simulink model "fromWorkSpace_TestGen6"  (R2017b)
settings: Solver=FixedStepDiscrete  StartTime=0.0  StopTime=10.0  RelTol=1e-3
model workspace (MAT data in the model file):
  X_matrix = [0 0.2 0.4 0.6 0.8 1 1.2 1.4 1.6 1.8 2 2.2 ... (200 elements, 50x4)]
undefined symbols (not defined in the file): Block_TestLib, trigger
settings Model: Creator=ktrinh  LastModifiedBy=ktrinh
settings DebuggingCC: ParameterOverflowMsg=none

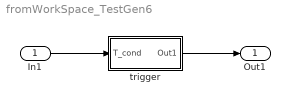
== system fromWorkSpace_TestGen6 ==
  In1 : Inport
  trigger : Subsystem  AncestorBlock=Block_TestLib/trigger
  Out1 : Outport
  wires:
  In1/1 -> trigger/1(T_cond)
  trigger/1(Out1) -> Out1/1

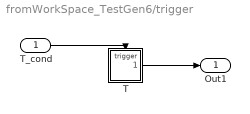
== system fromWorkSpace_TestGen6/trigger ==
  T_cond : Inport  OutDataTypeStr=boolean
  T : Subsystem  TreatAsAtomicUnit=on
  Out1 : Outport
  wires:
  T_cond/1 -> T/Trigger
  T/1(Out1) -> Out1/1

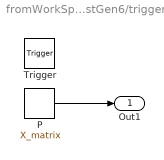
== system fromWorkSpace_TestGen6/trigger/T ==
  Trigger : TriggerPort  VariantControl=Variant
  P : FromWorkspace  VariableName=X_matrix  OutputAfterFinalValue=Holding final value
  Out1 : Outport
  wires:
  P/1 -> Out1/1
